simulink model "ar03_sim_RMNS"  (R2020a)
settings: Solver=ode45  StartTime=0.0  StopTime=55  RelTol=1e-3  EnableMultiTasking=on
values from neighbouring files (symbols this model uses):
  A = [1 0.3 0.2]    [ar03_spustima_RMNS.m]    (also in ar03_spustima_STR.m)
  B = [0 0.15]    [ar03_spustima_RMNS.m]    (also in ar03_spustima_STR.m)
  Tvz = 0.1    [ar03_spustima_RMNS.m]    (also in ar03_spustima_STR.m)
settings Model: Creator=MT  LastModifiedBy=MT
settings DataIOCC: LimitDataPoints=on  SaveFormat=Array  SignalLoggingSaveFormat=ModelDataLogs  SaveOutput=off  SignalLogging=off  SaveTime=off  ReturnWorkspaceOutputs=off
settings OptimizationCC: ExpressionDepthLimit=2147483647  InitFltsAndDblsToZero=on  LifeSpan=inf
settings DebuggingCC: SaveWithParameterizedLinksMsg=none  UnderspecifiedInitializationDetection=Classic  MergeDetectMultiDrivingBlocksExec=none  SignalResolutionControl=TryResolveAllWithWarning  SolverPrmCheckMsg=warning  MultiTaskDSMMsg=warning  MultiTaskCondExecSysMsg=none  FcnCallInpInsideContextMsg=warning  AllowSymbolicDim=off  StateNameClashWarn=warning  SFUnexpectedBacktrackingDiag=warning  SFNoUnconditionalDefaultTransitionDiag=warning  SFExecutionAtInitializationDiag=none  ArithmeticOperatorsInVariantConditions=warning
settings HardwareCC: ProdBitPerPointer=32  ProdBitPerSizeT=32  ProdBitPerPtrDiffT=32  ProdLargestAtomicFloat=None  ProdIntDivRoundTo=Undefined  ProdEndianess=Unspecified  ProdWordSize=32  ProdHWDeviceType=32-bit Generic
settings ModelReferenceCC: PropagateSignalLabelsOutOfModel=off
settings SFSimCC: SimUseLocalCustomCode=off  CustomCodeUndefinedFunction=UseInterfaceOnly
settings RTWCC: RTWUseLocalCustomCode=off
settings CodeAppCC: StateflowObjectComments=on
settings GRTTargetCC: TargetFcnLib=ansi_tfl_tmw.mat  TargetLangStandard=C89/C90 (ANSI)  CombineOutputUpdateFcns=off  GRTInterface=on
settings ConfigComp: CovMetricSettings=dw  CovHtmlReporting=on  CovSaveCumulativeToWorkspaceVar=on  CovSaveSingleToWorkspaceVar=on  CovExternalEMLEnable=off

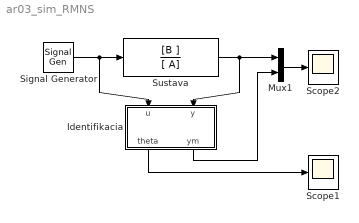
== system ar03_sim_RMNS ==
  Identifikacia : Subsystem
  Mux1 : Mux  Inputs=2
  Scope1 : Scope
  Scope2 : Scope
  Signal Generator : SignalGenerator  WaveForm=square  Amplitude=-1  Frequency=0.05
  Sustava : TransferFcn  Numerator=[B ]  Denominator=[ A]
  wires:
  Sustava/1 -> Mux1/1, Identifikacia/2(y)
  Signal Generator/1 -> Sustava/1, Identifikacia/1(u)
  Identifikacia/1(theta) -> Scope1/1
  Identifikacia/2(ym) -> Mux1/2
  Mux1/1 -> Scope2/1

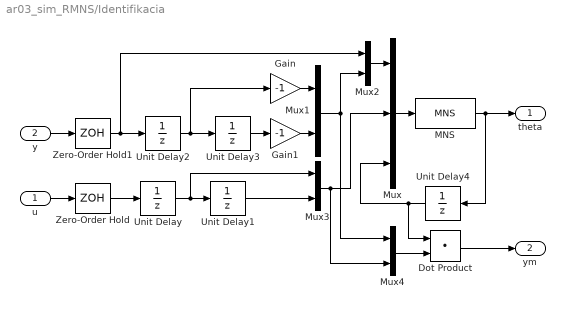
== system ar03_sim_RMNS/Identifikacia ==
  u : Inport
  y : Inport  Port=2
  Dot Product : DotProduct  InputSameDT=on  OutDataTypeStr=Inherit: Inherit via internal rule
  Gain : Gain  Gain=-1
  Gain1 : Gain  Gain=-1
  MNS : MATLABFcn  MATLABFcn=MNS  OutputDimensions=4
  Mux : Mux  Inputs=3
  Mux{1..4} (4 alike) : Mux  Inputs=2
  Unit Delay{,1..3} (4 alike) : UnitDelay  SampleTime=Tvz  HasFrameUpgradeWarning=on
  Unit Delay4 : UnitDelay  InitialCondition=[0.001 0.001 0.001 0.001]  SampleTime=Tvz  HasFrameUpgradeWarning=on
  Zero-Order Hold : ZeroOrderHold  SampleTime=Tvz
  Zero-Order Hold1 : ZeroOrderHold  SampleTime=Tvz
  theta : Outport
  ym : Outport  Port=2
  wires:
  u/1 -> Zero-Order Hold/1
  y/1 -> Zero-Order Hold1/1
  Zero-Order Hold/1 -> Unit Delay/1
  Unit Delay/1 -> Unit Delay1/1, Mux3/1
  Zero-Order Hold1/1 -> Unit Delay2/1, Mux2/1
  Unit Delay2/1 -> Unit Delay3/1, Gain/1
  Mux/1 -> MNS/1
  Unit Delay4/1 -> Mux/3, Dot Product/1
  Unit Delay1/1 -> Mux3/2
  Unit Delay3/1 -> Gain1/1
  Gain/1 -> Mux1/1
  Gain1/1 -> Mux1/2
  Mux1/1 -> Mux2/2, Mux4/1
  MNS/1 -> theta/1, Unit Delay4/1
  Dot Product/1 -> ym/1
  Mux2/1 -> Mux/1
  Mux3/1 -> Mux/2, Mux4/2
  Mux4/1 -> Dot Product/2
